simulink model "MKC_K9"  (R2025a)
settings: Solver=VariableStepAuto  StartTime=0.0  StopTime=30  MaxStep=2/50  RelTol=1e-3
settings Model: Creator=Szalay  LastModifiedBy=Szalay

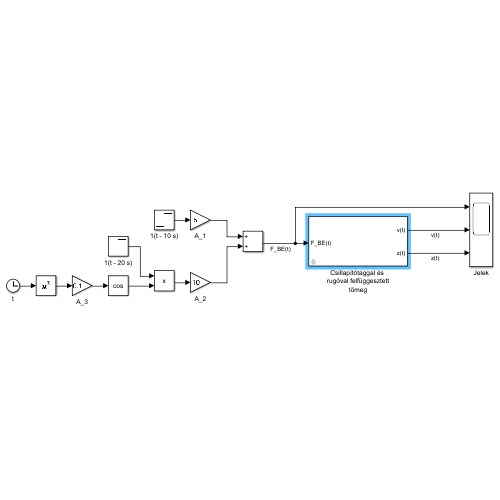
[thumbnail: Simulink's stored preview of the top-level diagram]
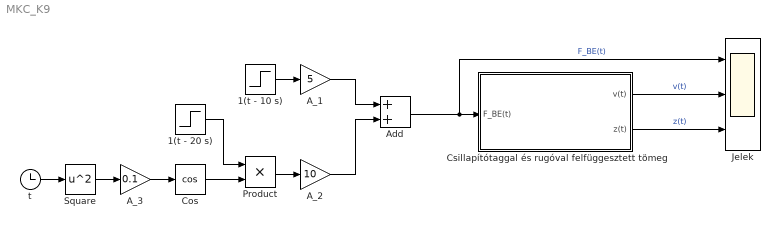
== system MKC_K9 ==
  1(t - 10 s) : Step  Time=10  SampleTime=0
  1(t - 20 s) : Step  Time=20  SampleTime=0
  A_1 : Gain  Gain=5
  A_2 : Gain  Gain=10
  A_3 : Gain  Gain=0.1
  Add : Sum
  Cos : Trigonometry  Operator=cos
  Csillapítótaggal és rugóval felfüggesztett tömeg : Subsystem  mask(Felfüggesztett rezgő tömeg){z_0=-0.1, v_0=-0.2, tau=2, xi=0.5, c=2}
      mask prompts: z_0 "Kezdeti elmozdulás (m)"; v_0 "Kezdeti sebesség (m/s)"; tau "Időállandó (s)"; xi "Csillapítási tényező"; c "Rugómerevség (N/m)"
      mask help: Csillapítótaggal és rugóval felfüggesztett tömeg rezgőmozgása.
      mask DialogControl ParameterGroupVar Prompt: Jellemzők
      mask DialogControl Container3 Prompt: Kezdeti értékek
  Jelek : Scope  NumInputPorts=3
      settings: ActiveDisplayYMinimum=-53.197495279178447  ActiveDisplayYMaximum=22.563537212639297
  Product : Product
  Square : Math  Operator=square
  t : Clock
  wires:
  Add/1 -> Jelek/1, Csillapítótaggal és rugóval felfüggesztett tömeg/1(F_BE(t))  "F_BE(t)"
  1(t - 10 s)/1 -> A_1/1
  A_1/1 -> Add/1
  A_2/1 -> Add/2
  Product/1 -> A_2/1
  1(t - 20 s)/1 -> Product/1
  Cos/1 -> Product/2
  A_3/1 -> Cos/1
  t/1 -> Square/1
  Square/1 -> A_3/1
  Csillapítótaggal és rugóval felfüggesztett tömeg/1(v(t)) -> Jelek/2  "v(t)"
  Csillapítótaggal és rugóval felfüggesztett tömeg/2(z(t)) -> Jelek/3  "z(t)"

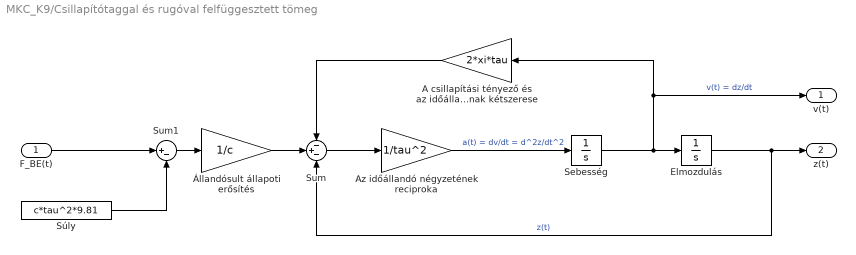
== system MKC_K9/Csillapítótaggal és rugóval felfüggesztett tömeg ==
  F_BE(t) : Inport
  A csillapítási tényező és az időállandó szorzatának kétszerese : Gain  Gain=2*xi*tau
  Az időállandó négyzetének reciproka : Gain  Gain=1/tau^2
  Elmozdulás : Integrator  InitialCondition=z_0
  Sebesség : Integrator  InitialCondition=v_0
  Sum : Sum  Inputs=-+-
  Sum1 : Sum  Inputs=|+-
  Súly : Constant  Value=c*tau^2*9.81
  Állandósult állapoti erősítés : Gain  Gain=1/c
  v(t) : Outport
  z(t) : Outport  Port=2
  wires:
  Állandósult állapoti erősítés/1 -> Sum/2
  Sebesség/1 -> v(t)/1, A csillapítási tényező és az időállandó szorzatának kétszerese/1, Elmozdulás/1  "v(t) = dz/dt"
  F_BE(t)/1 -> Sum1/1
  Elmozdulás/1 -> z(t)/1, Sum/3  "z(t)"
  Sum/1 -> Az időállandó négyzetének reciproka/1
  A csillapítási tényező és az időállandó szorzatának kétszerese/1 -> Sum/1
  Az időállandó négyzetének reciproka/1 -> Sebesség/1  "a(t) = dv/dt = d^2z/dt^2"
  Sum1/1 -> Állandósult állapoti erősítés/1
  Súly/1 -> Sum1/2
